simulink model "AutonomousScan"  (R2019a)
settings: Solver=FixedStepAuto  StartTime=0.0  StopTime=inf  FixedStep=0.001  RelTol=1e-3
libraries: dspnetwork x24, simulink_extras x3, etargetslib x1, dspmtrx3 x1, dspstat3 x1, simulink x1
(part 1 of 2)
settings Model: EnablePacing=on  Creator=jakub  LastModifiedBy=kirill
settings SolverCC: AutoInsertRateTranBlk=on
settings DataIOCC: ReturnWorkspaceOutputs=off
settings HardwareCC: ProdBitPerLong=64  ProdHWDeviceType=Intel->x86-64 (Linux 64)

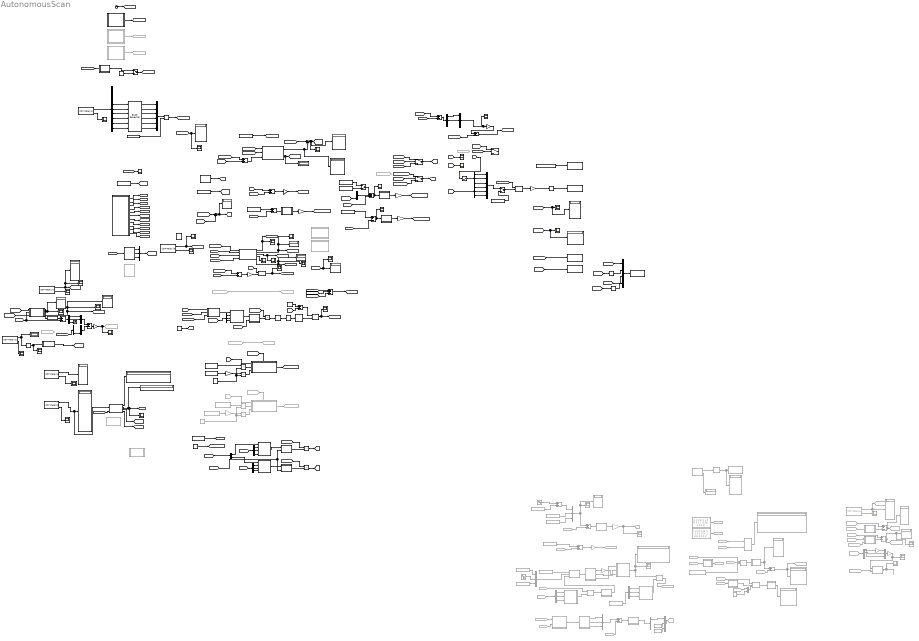
== system AutonomousScan ==
  note: Experimental RCM based on frame transforms - does not work. See ipad notes for details
  note: Experimental RCM based on screw axis - does not work
  note: Motoman - receiver (temp)
  note: Motoman Joint Position Control - depracated
  note: position control and trajectory generation
  note: force control
  note: y and z axes are zero'd twice (matlab function and matrix multiplication)
  note: transforms force sensor measured force to panda end effector frame to base frame
  note: Biasing sensor and panda position before moving - incorrect approach
  Add1 : Sum  Inputs=++-
  Add2 : Sum  Inputs=+-
  Add3 : Sum  Inputs=+-
  Byte Reversal : etargetslib/Byte Reversal  numInp=6
      settings: SourceProductName=MATLAB Coder  SourceProductBaseCode=ME
  Clock : Clock
  Constant1 : Constant  Commented=on  Value=[0.45;0;0.3]
  Constant10 : Constant  Value=[0.45;0;0.45]
  Constant11 : Constant  Value=0.25
  Constant12 : Constant  Value=[0;0;0]
  Constant13 : Constant  Value=2.25
  Constant14 : Constant  Value=-1.4
  Constant15 : Constant  Commented=on  Value=[0.25;0.25;0.25]
  Constant16 : Constant  Commented=on  Value=[0.5;0.5;0.5]
  Constant17 : Constant  Commented=on  Value=[0]
  Constant18 : Constant  Value=[0.553;0;0]
  Constant19 : Constant  Commented=on  Value=[0.5 0 0.06]
  Constant2 : Constant  Value=8.295632e-317  OutDataTypeStr=double
  Constant20 : Constant  Commented=on  Value=3.14
  Constant21 : Constant  Commented=on  Value=[0.5]
  Constant22 : Constant
  Constant23 : Constant  Value=1000000
  Constant24 : Constant  Value=[pi;0;-0.2]
  Constant25 : Constant  Commented=on  Value=[ 0.03]
  Constant26 : Constant  Commented=on  Value=[0]
  Constant27 : Constant  Commented=on  Value=[ 0]
  Constant28 : Constant  Commented=on  Value=[0;-pi;pi/2]
  Constant29 : Constant  Commented=on  Value=[0;0;0.02;1]
  Constant3 : Constant  Value=[0;0;0;0;0;0]
  Constant30 : Constant  Commented=on  Value=[1 0 0 0; 0 1 0 0; 0 0 1 -0.05; 0 0 0 1]
  Constant31 : Constant  Commented=on  Value=[1]
  Constant32 : Constant  Commented=on  Value=[1 0 0 0.45; 0 -1 0 0; 0 0 -1 0.3; 0 0 0 1]
  Constant33 : Constant  Value=[pi;0;pi/2-0.2]
  Constant34 : Constant  Value=[pi;0;-0.2]
  Constant35 : Constant  Value=[pi;0;-0.2]
  Constant4 : Constant  Value=[1 0 0; 0 1 0; 0 0 0]
  Constant5 : Constant  Commented=on  Value=[0]
  Constant6 : Constant  Value=[pi/2;0;pi]
  Constant7 : Constant  Commented=on  Value=1.5
  Constant8 : Constant  Value=[2.5;2.5;2.5]
  Constant9 : Constant  Value=[5;5;5]
  Degrees to Radians : simulink_extras/Transformations/Degrees to Radians
  Demux{1..2,4..5,7,12..13,15} (8 alike) : Demux  Outputs=3
  Demux10 : Demux  Commented=on  Outputs=7
  Demux11 : Demux  Outputs=9
  Demux3 : Demux  Outputs=2
  Demux6 : Demux  Commented=on  Outputs=3
  Demux8 : Demux  Commented=on  Outputs=3
  Demux9 : Demux  Commented=on  Outputs=3
  DerivOut1 : Scope
  Display{1..6,9..10,12,21..29} (18 alike) : Display
      Display2 settings: Decimation=4
      Display3 settings: Decimation=4
      Display4 settings: Decimation=4
  Display{7..8,11,13..20} (11 alike) : Display  Commented=on
      Display13 settings: Decimation=4
      Display14 settings: Decimation=4
      Display16 settings: Decimation=4
  Divide4 : Product  Inputs=*/  OutDataTypeStr=double
  From1 : From  Commented=on  GotoTag=M_cart
  From12 : From  Commented=on  GotoTag=admission_vel_cart
  From26 : From  Commented=on  GotoTag=bias_good
  From30 : From  Commented=on  GotoTag=admission_vel_rot
  From47 : From  Commented=on  GotoTag=vel_rot
  From48 : From  Commented=on  GotoTag=panda_pos_biased
  From49 : From  Commented=on  GotoTag=sensor
  From50 : From  Commented=on  GotoTag=sensor
  From51 : From  Commented=on  GotoTag=scan_complete
  From{52..53,57,68,70,74} (6 alike) : From  Commented=on  GotoTag=panda_pos
  From55 : From  Commented=on  GotoTag=panda_rpy
  From58 : From  Commented=on  GotoTag=panda_so3
  From60 : From  Commented=on  GotoTag=axia_ft
  From61 : From  Commented=on  GotoTag=rot_des_bf2
  From62 : From  Commented=on  GotoTag=panda_so3
  From63 : From  Commented=on  GotoTag=panda_so3
  From64 : From  Commented=on  GotoTag=panda_rpy
  From65 : From  Commented=on  GotoTag=T_B_EE
  From67 : From  Commented=on  GotoTag=T_U_EE
  From71 : From  Commented=on  GotoTag=invU
  From72 : From  Commented=on  GotoTag=T_U_EE
  From73 : From  Commented=on  GotoTag=T_B_EE
  From75 : From  Commented=on  GotoTag=sensor_biased
  From80 : From  Commented=on  GotoTag=bias_good
  From90 : From  Commented=on  GotoTag=admission_control
  Gain : Gain  Gain=3.0
  Gain1 : Gain  Gain=2.5
  Gain10 : Gain  Commented=on  Gain=-1
  Gain11 : Gain  Gain=3.0
  Gain{4..5,12,14} (4 alike) : Gain  Gain=0.5
  Gain13 : Gain  Gain=3.0
  Gain2 : Gain  Gain=1.0
  Gain3 : Gain  Commented=on  Gain=2.75
  Gain6 : Gain  Commented=on  Gain=0.5
  Gain7 : Gain  Commented=on  Gain=3.0
  Gain8 : Gain  Commented=on  Gain=0
  Gain9 : Gain  Commented=on  Gain=0.1
  Goto13 : Goto  Commented=on  GotoTag=admission_vel_rot
  Goto17 : Goto  Commented=on  GotoTag=admission_control
  Goto27 : Goto  Commented=on  GotoTag=sensor
  Goto28 : Goto  Commented=on  GotoTag=vel_rot
  Goto29 : Goto  Commented=on  GotoTag=sensor_biased
  Goto30 : Goto  Commented=on  GotoTag=panda_pos_biased
  Goto31 : Goto  Commented=on  GotoTag=V_cart_2
  Goto32 : Goto  Commented=on  GotoTag=vel_rot
  Goto33 : Goto  Commented=on  GotoTag=vel_tran_temp
  Goto34 : Goto  Commented=on  GotoTag=rot_des_bf2
  Goto36 : Goto  Commented=on  GotoTag=vel_rot
  Goto41 : Goto  Commented=on  GotoTag=vel_tran_temp
  Goto42 : Goto  Commented=on  GotoTag=panda_ijac
  Goto43 : Goto  Commented=on  GotoTag=panda_state
  Goto47 : Goto  Commented=on  GotoTag=invU
  Goto48 : Goto  Commented=on  GotoTag=T_U_EE
  Goto57 : Goto  Commented=on  GotoTag=T_B_EE
  Identity Matrix : dspmtrx3/Identity Matrix  Inherit=off  N=3  Ts=1  dataType=double  isSigned=on  wordLen=16  udDataType=sfix(16)  fracBitsMode=Best precision  numFracBits=15  OutDataTypeStr=double  LastOutDataTypeStr=double
      settings: SourceProductName=DSP System Toolbox
  MATLAB Function : MATLAB Function  TreatAsAtomicUnit=on
  MATLAB Function1 : MATLAB Function  TreatAsAtomicUnit=on
  MATLAB Function10 : MATLAB Function  Commented=on  TreatAsAtomicUnit=on
  MATLAB Function11 : MATLAB Function  Commented=on  TreatAsAtomicUnit=on
  MATLAB Function12 : MATLAB Function  Commented=on  TreatAsAtomicUnit=on
  MATLAB Function13 : MATLAB Function  Commented=on  TreatAsAtomicUnit=on
  MATLAB Function14 : MATLAB Function  Commented=on  TreatAsAtomicUnit=on
  MATLAB Function15 : MATLAB Function  Commented=on  TreatAsAtomicUnit=on
  MATLAB Function16 : MATLAB Function  Commented=on  TreatAsAtomicUnit=on
  MATLAB Function17 : MATLAB Function  Commented=on  TreatAsAtomicUnit=on
  MATLAB Function18 : MATLAB Function  Commented=on  TreatAsAtomicUnit=on
  MATLAB Function19 : MATLAB Function  Commented=on  TreatAsAtomicUnit=on
  MATLAB Function2 : MATLAB Function  TreatAsAtomicUnit=on
  MATLAB Function20 : MATLAB Function  Commented=on  TreatAsAtomicUnit=on
  MATLAB Function21 : MATLAB Function  Commented=on  TreatAsAtomicUnit=on
  MATLAB Function22 : MATLAB Function  Commented=on  TreatAsAtomicUnit=on
  MATLAB Function23 : MATLAB Function  Commented=on  TreatAsAtomicUnit=on
  MATLAB Function24 : MATLAB Function  Commented=on  TreatAsAtomicUnit=on
  MATLAB Function25 : MATLAB Function  Commented=on  TreatAsAtomicUnit=on
  MATLAB Function26 : MATLAB Function  TreatAsAtomicUnit=on
  MATLAB Function27 : MATLAB Function  TreatAsAtomicUnit=on
  MATLAB Function28 : MATLAB Function  TreatAsAtomicUnit=on
  MATLAB Function29 : MATLAB Function  Commented=on  TreatAsAtomicUnit=on
  MATLAB Function3 : MATLAB Function  TreatAsAtomicUnit=on
  MATLAB Function30 : MATLAB Function  TreatAsAtomicUnit=on
  MATLAB Function31 : MATLAB Function  Commented=on  TreatAsAtomicUnit=on
  MATLAB Function32 : MATLAB Function  TreatAsAtomicUnit=on
  MATLAB Function33 : MATLAB Function  TreatAsAtomicUnit=on
  MATLAB Function34 : MATLAB Function  TreatAsAtomicUnit=on
  MATLAB Function4 : MATLAB Function  TreatAsAtomicUnit=on
  MATLAB Function5 : MATLAB Function  TreatAsAtomicUnit=on
  MATLAB Function6 : MATLAB Function  TreatAsAtomicUnit=on
  MATLAB Function7 : MATLAB Function  TreatAsAtomicUnit=on
  MATLAB Function8 : MATLAB Function  TreatAsAtomicUnit=on
  MATLAB Function9 : MATLAB Function  Commented=on  TreatAsAtomicUnit=on
  Manual Switch : ManualSwitch
  Manual Switch1 : ManualSwitch  CurrentSetting=0
  Matrix Multiply : Product  Multiplication=Matrix(*)
  Matrix Multiply1 : Product  Multiplication=Matrix(*)
  Matrix Multiply2 : Product  Multiplication=Matrix(*)
  Matrix Multiply3 : Product  Commented=on  Multiplication=Matrix(*)
  Matrix Multiply4 : Product  Commented=on  Multiplication=Matrix(*)
  Matrix Multiply5 : Product  Commented=on  Inputs=3  Multiplication=Matrix(*)
  Matrix Multiply6 : Product  Commented=on  Inputs=3  Multiplication=Matrix(*)
  Moving Average : dspstat3/Moving Average  Method=Sliding window  ForgettingFactorPort=off  SpecifyWindowLength=on  WindowLength=800  ForgettingFactor=0.9  SimulateUsing=Code generation
  Mux : Mux  Inputs=6
  Mux{1..4,6} (5 alike) : Mux  Commented=on  Inputs=3
  Mux10 : Mux  Inputs=6
  Mux11 : Mux
  Mux{7..9,12,14} (5 alike) : Mux  Inputs=3
  Mux5 : Mux  Commented=on  Inputs=2
  NetworkPacket : Scope
  New Phantom : MATLAB Function  TreatAsAtomicUnit=on
  PID Controller2 : simulink/Continuous/PID Controller  Controller=PID  Form=Parallel  TimeDomain=Continuous-time  SampleTime=-1  IntegratorMethod=Forward Euler  FilterMethod=Forward Euler  ControllerParametersSource=internal  P=0.2  I=0  D=0.1  UseFilter=on  N=100  TunerSelectOption=Transfer Function Based (PID Tuner App)  InitialConditionSource=internal  InitialConditionForIntegrator=0  InitialConditionForFilter=0  DifferentiatorICPrevScaledInput=0  ExternalReset=none  TrackingMode=off  Kt=1  LimitOutput=off  UpperSaturationLimit=inf  LowerSaturationLimit=-inf  LinearizeAsGain=on  AntiWindupMode=none  Kb=1  POutMin=[]  POutMax=[]  IOutMin=[]  IOutMax=[]  DOutMin=[]  DOutMax=[]  NOutMin=[]  NOutMax=[]  SumOutMin=[]  SumOutMax=[]  SaturationOutMin=[]  SaturationOutMax=[]  PParamMin=[]  PParamMax=[]  IParamMin=[]  IParamMax=[]  DParamMin=[]  DParamMax=[]  NParamMin=[]  NParamMax=[]  KbParamMin=[]  KbParamMax=[]  KtParamMin=[]  KtParamMax=[]  KbOutMin=[]  KbOutMax=[]  KtOutMin=[]  KtOutMax=[]  IntegratorOutMin=[]  IntegratorOutMax=[]  FilterOutMin=[]  FilterOutMax=[]  SumI1OutMin=[]  SumI1OutMax=[]  SumI2OutMin=[]  SumI2OutMax=[]  SumI3OutMin=[]  SumI3OutMax=[]  SumI4OutMin=[]  SumI4OutMax=[]  SumDOutMin=[]  SumDOutMax=[]  DifferentiatorOutMin=[]  DifferentiatorOutMax=[]  FilterDiffOutCoefMin=[]  FilterDiffOutCoefMax=[]  ReciprocalOutMin=[]  ReciprocalOutMax=[]  SumDenOutMin=[]  SumDenOutMax=[]  SumNumOutMin=[]  SumNumOutMax=[]  DivideOutMin=[]  DivideOutMax=[]  IntegratorContinuousStateAttributes=''  IntegratorStateMustResolveToSignalObject=off  IntegratorRTWStateStorageClass=Auto  FilterContinuousStateAttributes=''  FilterStateMustResolveToSignalObject=off  FilterRTWStateStorageClass=Auto  ParallelPVariant=InternalParameters  IdealPVariant=Disabled  IVariant=InternalParameters  DVariant=InternalParameters  IntegratorVariant=Continuous  SatVariant=Disabled  AWVariant=Passthrough  PCopyVariant=Disabled  TRVariant=Disabled  FdbkBlocksVariant=Forward  IdealPFdbkVariant=Disabled  SatFdbkVariant=Disabled  DerivativeFilterVariant=ContFilter  NVariant=InternalParameters  NCopyVariant=Disabled  FilterICVariant=InternalICsFilter  IntegratorICVariant=InternalICs  ExternalResetVariant=Disabled  TRSumVariant=Passthrough  SumFdbkVariant=Disabled  SumVariant=Sum_PID
  PandaPosition : Scope
  PandaRotation : Scope
  PandaRotation1 : Scope  Commented=on
  Panda_inv_jac_receive : Subsystem  Commented=on
  Panda_inv_jac_receive1 : Subsystem  Commented=on
  Product{,1,4..6} (5 alike) : Product
  Product2 : Product  Commented=on
  Product3 : Product  Commented=on
  Radians to Degrees : simulink_extras/Transformations/Radians to Degrees
  Radians to Degrees1 : simulink_extras/Transformations/Radians to Degrees
  Rate Limiter1 : RateLimiter  RisingSlewLimit=2.0  FallingSlewLimit=-2.0  SampleTimeMode=inherited
  Rate Limiter3 : RateLimiter  RisingSlewLimit=0.15  FallingSlewLimit=-0.15  SampleTimeMode=inherited
  Rate Transition : RateTransition  OutPortSampleTime=0.01
  Rate Transition1 : RateTransition  Commented=on  OutPortSampleTime=2
  STOP_SWITCH1 : ManualSwitch
  Saturation : Saturate  UpperLimit=0.1  LowerLimit=-0.1
  Scope{,1..9,12,17..23,25..26,28..29} (22 alike) : Scope
  Scope{10..11,13..16} (6 alike) : Scope  Commented=on
  Sine Wave : Sin  Commented=on  Amplitude=0.4  Frequency=3  SampleTime=0
  Sine Wave1 : Sin  Commented=on  Amplitude=0.05  Frequency=3  SampleTime=0
  Subtract{1..4,13,15..16} (7 alike) : Sum  Inputs=+-
  Subtract10 : Sum  Commented=on
  Subtract{5..8,11..12} (6 alike) : Sum  Commented=on  Inputs=+-
  Subtract14 : Sum  Inputs=+--
  Subtract9 : Sum
  Sum : Sum  Inputs=|+-
  Sum2 : Sum  Inputs=|++
  Switch1 : Switch  Criteria=u2 > Threshold
  Switch2 : Switch  Criteria=u2 > Threshold
  Switch3 : Switch  Criteria=u2 > Threshold
  Terminator : Terminator
  Trajectory Generation (works) : MATLAB Function  Commented=on  TreatAsAtomicUnit=on
  Trajectory Generation1 : MATLAB Function  Commented=on  TreatAsAtomicUnit=on
  UDP Receive1 : dspnetwork/UDP Receive  localURL='0.0.0.0'  localPort=49154  remoteURL='192.168.0.13'  remotePort=-1  recvBufferSize=36  dims=9  signalDatatype=int32  isComplex=off  isVarSize=off  showBlockingTime=off  blockingTime=0  sampletime=0.001  blockPlatform=[]
      settings: SourceProductName=Simulink
  UDP Receive2 : dspnetwork/UDP Receive  localURL='0.0.0.0'  localPort=25010  remoteURL='10.1.38.120'  remotePort=-1  recvBufferSize=8192  dims=1  signalDatatype=double  isComplex=off  isVarSize=off  showBlockingTime=off  blockingTime=0  sampletime=0.001  blockPlatform=[]
      settings: SourceProductName=Simulink
  UDP Receive3 : dspnetwork/UDP Receive  Commented=on  localURL='0.0.0.0'  localPort=1502  remoteURL='10.1.38.120'  remotePort=-1  recvBufferSize=8192  dims=7  signalDatatype=double  isComplex=off  isVarSize=off  showBlockingTime=off  blockingTime=0  sampletime=0.001  blockPlatform=[]
      settings: SourceProductName=Simulink
  UDP Receive4 : dspnetwork/UDP Receive  localURL='0.0.0.0'  localPort=30011  remoteURL='0.0.0.0'  remotePort=-1  recvBufferSize=8192  dims=7  signalDatatype=double  isComplex=off  isVarSize=off  showBlockingTime=off  blockingTime=0  sampletime=0.1  blockPlatform=[]
      settings: SourceProductName=Simulink
  UDP Receive5 : dspnetwork/UDP Receive  localURL='0.0.0.0'  localPort=1502  remoteURL='192.168.100.101'  remotePort=-1  recvBufferSize=8192  dims=7  signalDatatype=double  isComplex=off  isVarSize=off  showBlockingTime=off  blockingTime=0  sampletime=0.001  blockPlatform=[]
      settings: SourceProductName=Simulink
  UDP Receive6 : dspnetwork/UDP Receive  localURL='0.0.0.0'  localPort=30015  remoteURL='0.0.0.0'  remotePort=-1  recvBufferSize=8192  dims=15  signalDatatype=double  isComplex=off  isVarSize=off  showBlockingTime=off  blockingTime=0  sampletime=0.1  blockPlatform=[]
      settings: SourceProductName=Simulink
  UDP Receive7 : dspnetwork/UDP Receive  localURL='0.0.0.0'  localPort=1508  remoteURL='10.1.38.120'  remotePort=-1  recvBufferSize=8192  dims=1  signalDatatype=double  isComplex=off  isVarSize=off  showBlockingTime=off  blockingTime=0  sampletime=0.001  blockPlatform=[]
      settings: SourceProductName=Simulink
  UDP Send1 : dspnetwork/UDP Send  remoteURL='127.0.0.1'  remotePort=39474  localURL='0.0.0.0'  localPortSource=Automatically determine  localPort=48000  sampletime=-1  blockPlatform=[]  separateLengthPort=0
      settings: SourceProductName=Simulink
  UDP Send2 : dspnetwork/UDP Send  remoteURL='10.1.38.120'  remotePort=25002  localURL='0.0.0.0'  localPortSource=Specify via dialog  localPort=25004  sampletime=-1  blockPlatform=[]  separateLengthPort=0
      settings: SourceProductName=Simulink
  UDP Send3 : dspnetwork/UDP Send  remoteURL='10.1.38.120'  remotePort=25006  localURL='0.0.0.0'  localPortSource=Specify via dialog  localPort=25008  sampletime=-1  blockPlatform=[]  separateLengthPort=0
      settings: SourceProductName=Simulink
  UDP Send4 : dspnetwork/UDP Send  remoteURL='192.168.0.13'  remotePort=49152  localURL='0.0.0.0'  localPortSource=Specify via dialog  localPort=49154  sampletime=-1  blockPlatform=[]  separateLengthPort=0
      settings: SourceProductName=Simulink
  UDP Send5 : dspnetwork/UDP Send  Commented=on  remoteURL='127.0.0.1'  remotePort=39575  localURL='0.0.0.0'  localPortSource=Automatically determine  localPort=48000  sampletime=-1  blockPlatform=[]  separateLengthPort=0
      settings: SourceProductName=Simulink
  UDP Send6 : dspnetwork/UDP Send  remoteURL='10.1.38.120'  remotePort=35000  localURL='0.0.0.0'  localPortSource=Specify via dialog  localPort=25008  sampletime=-1  blockPlatform=[]  separateLengthPort=0
      settings: SourceProductName=Simulink
  Velocity Controller1 : Subsystem
  Velocity Controller2 : Subsystem  Commented=on
  VelocityOut{,1..4} (5 alike) : Scope
  in general1 : MATLAB Function  TreatAsAtomicUnit=on
  in general2 : MATLAB Function  Commented=on  TreatAsAtomicUnit=on
  in general3 : MATLAB Function  Commented=on  TreatAsAtomicUnit=on
  in general4 : MATLAB Function  Commented=on  TreatAsAtomicUnit=on
  joy_state_receive1 : Subsystem
  panda_data_receive : Subsystem
  wires:
  Demux2/1 -> Mux/1
  Demux1/2 -> Mux/5
  Demux1/1 -> Mux/4
  Demux2/2 -> Mux/2
  Demux1/3 -> Mux/6
  Demux2/3 -> Mux/3
  [V_rot] -> Demux1/1
  Constant18/1 -> [P_tissue]
  joy_state_receive1/1("joy_state ") -> [joy_state]
  Panda_inv_jac_receive1/1(panda_state) -> Goto43/1
  [joy_state] -> MATLAB Function33/1(u)
  MATLAB Function33/1(stop) -> STOP_SWITCH1/1
  Panda_inv_jac_receive/1(inverse_jacobian) -> Goto42/1
  STOP_SWITCH1/1 -> [stop_manual]
  Constant22/1 -> STOP_SWITCH1/2
  in general1/1(grad) -> Mux7/1
  in general1/2(brad) -> Mux7/2
  in general1/3(arad) -> Mux7/3
  Mux7/1 -> [panda_rpy]
  [panda_ijac] -> Matrix Multiply/1
  Clock/1 -> [sim_time]
  UDP Receive1/2 -> NetworkPacket/1
  Byte Reversal/4 -> Mux10/4
  Divide4/1 -> [axia_force]
  Byte Reversal/2 -> Mux10/2
  Constant23/1 -> Divide4/2
  Demux11/7 -> Byte Reversal/4
  Mux10/1 -> Divide4/1
  Byte Reversal/1 -> Mux10/1
  Demux11/5 -> Byte Reversal/2
  UDP Receive1/1 -> Demux11/1
  Demux11/6 -> Byte Reversal/3
  Byte Reversal/3 -> Mux10/3
  Demux11/9 -> Byte Reversal/6
  Demux11/8 -> Byte Reversal/5
  Demux11/4 -> Byte Reversal/1
  Byte Reversal/5 -> Mux10/5
  Byte Reversal/6 -> Mux10/6
  [panda_pos] -> Display4/1, PandaPosition/1
  [V_cart] -> VelocityOut/1
  panda_data_receive/9(panda_tau) -> [panda_tau]
  panda_data_receive/4(panda_force) -> [panda_force]
  panda_data_receive/2(panda_pos) -> [panda_pos]
  panda_data_receive/10(panda_state) -> [panda_state]
  panda_data_receive/3(panda_so3) -> [panda_so3]
  panda_data_receive/7(inverse_jacobian) -> [panda_ijac]
  panda_data_receive/6(panda_dq) -> [panda_dq]
  panda_data_receive/1(ros_time) -> [ros_time]
  panda_data_receive/5(panda_q) -> [panda_q]
  panda_data_receive/8(jacobian) -> [panda_jac]
  [panda_rpy] -> Display3/1, PandaRotation/1
  Constant24/1 -> Subtract3/1
  [panda_rpy] -> Subtract3/2
  panda_data_receive/11(networkVals) -> [networkVals]
  [p_des] -> Subtract1/1
  Gain2/1 -> Rate Limiter1/1
  Matrix Multiply/1 -> Gain2/1
  Constant2/1 -> UDP Send4/1
  Subtract1/1 -> Gain/1
  [panda_pos] -> Subtract1/2
  [panda_ijac] -> DerivOut1/1
  Sum2/1 -> Display1/1, [p_des]
  [probe_offset] -> Sum2/2
  Saturation/1 -> Demux2/1
  Constant12/1 -> [probe_offset]
  Mux/1 -> Manual Switch/1
  Manual Switch/1 -> Matrix Multiply/2
  Constant3/1 -> Manual Switch/2
  [axia_force] -> Scope5/1, Display2/1
  MATLAB Function5/1(bias) -> Display6/1, Sum/2
  [axia_force] -> Sum/1
  Sum/1 -> Scope/1, Display10/1, [axia_biased]
  MATLAB Function5/2(forceBiasGood) -> Display5/1, [bias_good]
  Constant10/1 -> [p_bias]
  [axia_force] -> MATLAB Function5/1(forceMeasure)
  [p_bias] -> Subtract9/1
  Constant11/1 -> [f_scale_factor]
  MATLAB Function8/1(x_rot) -> Product5/2
  MATLAB Function/1(x_rot) -> Product4/2
  Demux3/2 -> MATLAB Function7/1(X)
  Demux4/2 -> MATLAB Function7/3(brad)
  Demux5/3 -> MATLAB Function6/4(grad)
  Demux3/1 -> MATLAB Function6/1(X)
  [axia_ft] -> Demux5/1
  Demux4/3 -> MATLAB Function7/4(grad)
  Demux4/1 -> MATLAB Function7/2(arad)
  [axia_ft] -> Demux4/1
  MATLAB Function6/1(X_t) -> MATLAB Function/1(x)
  [f_scale_factor] -> Product5/1
  [f_scale_factor] -> Product4/1
  Product4/1 -> [F_cart]
  MATLAB Function7/1(X_t) -> MATLAB Function8/1(x)
  [panda_so3] -> MATLAB Function/2(R), MATLAB Function8/2(R)
  Demux5/2 -> MATLAB Function6/3(brad)
  Product5/1 -> [M_cart]
  Constant6/1 -> [axia_ft]
  Gain1/1 -> Product1/1
  Constant8/1 -> Product/1
  Constant9/1 -> Gain1/1
  Product/1 -> Velocity Controller1/2(m)
  Product1/1 -> Velocity Controller1/3(c)
  [F_cart] -> Velocity Controller1/1(F_Total)
  [bias_good] -> Switch1/2
  [p_bias] -> Sum2/1
  Demux5/1 -> MATLAB Function6/2(arad)
  Constant13/1 -> Product1/2, Product/2
  [V_rot] -> VelocityOut1/1
  Gain3/1 -> Product3/1
  Product3/1 -> Velocity Controller2/3(c)
  Constant7/1 -> Product2/2, Product3/2
  Constant16/1 -> Gain3/1
  Product2/1 -> Velocity Controller2/2(m)
  Constant15/1 -> Product2/1
  From1/1 -> Velocity Controller2/1(M_Total)
  [bias_good] -> Switch3/2
  Switch3/1 -> [V_rot]
  [bias_good] -> Velocity Controller1/Enable
  [initial_vel_rot] -> Switch3/3
  From26/1 -> Velocity Controller2/Enable
  Velocity Controller2/1(Vel_Rot) -> Goto13/1
  [initial_vel_tran] -> Switch1/3
  [vel_rot_scan] -> Switch3/1
  Rate Limiter1/1 -> UDP Send1/1
  From30/1 -> Goto28/1
  [vel_tran] -> Switch1/1
  Switch1/1 -> [V_cart]
  Subtract3/1 -> MATLAB Function1/1(u)
  Gain/1 -> [initial_vel_tran]
  MATLAB Function1/1(y) -> Gain5/1
  Gain5/1 -> [initial_vel_rot]
  [panda_pos] -> Subtract2/2
  Constant14/1 -> [fdes_z]
  [axia_biased] -> Demux3/1
  Velocity Controller1/1(Vel_Cart) -> [admission_vel_cart]
  [fdes_z] -> MATLAB Function3/1(f_des)
  [axia_biased] -> MATLAB Function3/2(f_act)
  [bias_good] -> MATLAB Function3/3(bias_good)
  Demux7/1 -> MATLAB Function4/2(arad)
  Demux7/2 -> MATLAB Function4/3(brad)
  [panda_so3] -> MATLAB Function2/2(R)
  MATLAB Function4/1(X_t) -> MATLAB Function2/1(x)
  MATLAB Function2/1(x_rot) -> Product6/2
  Demux7/3 -> MATLAB Function4/4(grad)
  [axia_ft] -> Demux7/1
  MATLAB Function3/1(f_err) -> MATLAB Function4/1(X)
  [f_scale_factor] -> Product6/1
  PID Controller2/1 -> Rate Limiter3/1
  Matrix Multiply1/1 -> Scope4/1, [pos_control]
  Constant4/1 -> [S]
  Identity Matrix/1 -> Subtract4/1
  [S] -> Subtract4/2
  Subtract4/1 -> Matrix Multiply2/1
  Product6/1 -> PID Controller2/1
  Rate Limiter3/1 -> Moving Average/1
  [S] -> Matrix Multiply1/1
  Matrix Multiply2/1 -> [force_control], Scope2/1
  Moving Average/1 -> Matrix Multiply2/2
  From12/1 -> Goto17/1
  [admission_control] -> Add1/2
  [force_control] -> Add1/3
  [pos_des] -> Subtract2/1
  [panda_pos] -> New Phantom/2(current_pos)
  New Phantom/1(pos_des) -> [pos_des], Scope1/1
  New Phantom/2(record_data) -> Scope6/1, Display9/1, [record_data]
  [axia_biased] -> New Phantom/3(measured_force)
  [bias_good] -> New Phantom/4(bias_good)
  Subtract2/1 -> Gain4/1
  [shutter] -> UDP Send2/1
  [panda_pos] -> UDP Send3/1
  Gain4/1 -> Matrix Multiply1/2
  New Phantom/3(shutter) -> Scope3/1, [shutter]
  UDP Receive2/2 -> Scope7/1
  [shutter_fb] -> New Phantom/1(shutter_fb)
  New Phantom/4(pnts) -> Scope9/1
  UDP Receive4/1 -> Display12/1
  UDP Receive4/2 -> Scope12/1
  Rate Transition1/1 -> Display13/1, UDP Send5/1
  MATLAB Function12/1(y) -> Rate Transition1/1
  MATLAB Function12/2(limit) -> Display14/1
  Subtract10/1 -> Mux1/1
  Constant5/1 -> Mux1/2
  Constant17/1 -> Mux1/3
  MATLAB Function13/1(y) -> Gain6/1
  Gain6/1 -> Scope14/1, Goto32/1
  [panda_pos] -> MATLAB Function5/2(currentPos)
  Subtract9/1 -> MATLAB Function5/3(desiredPos)
  [probe_offset] -> Subtract9/2
  Sine Wave/1 -> Subtract10/1
  Constant20/1 -> Subtract10/2
  Subtract7/1 -> MATLAB Function13/1(u)
  Mux1/1 -> Scope13/1, Display17/1, Subtract7/1
  From55/1 -> Subtract7/2
  [panda_so3] -> in general1/1(R)
  Constant1/1 -> Subtract11/1
  Subtract11/1 -> Gain7/1
  From57/1 -> Subtract11/2
  Gain7/1 -> Goto33/1
  Constant19/1 -> MATLAB Function14/1(rcm)
  Mux3/1 -> MATLAB Function14/2(tip)
  MATLAB Function14/1(rotmat) -> in general3/1(R)
  in general3/1(grad) -> Gain8/1
  in general3/2(brad) -> MATLAB Function15/2(brad)
  in general3/3(arad) -> MATLAB Function15/1(arad)
  Gain8/1 -> MATLAB Function15/3(grad)
  From60/1 -> Demux6/1
  From58/1 -> Matrix Multiply3/1
  MATLAB Function16/1(R) -> Matrix Multiply3/2
  Matrix Multiply3/1 -> MATLAB Function17/1(u)
  MATLAB Function17/1(y) -> MATLAB Function14/3(currentZ)
  Constant28/1 -> Demux8/1
  MATLAB Function15/1(R) -> Display16/1, PandaRotation1/1, Matrix Multiply4/1
  MATLAB Function18/1(R) -> Matrix Multiply4/2
  Matrix Multiply4/1 -> Goto34/1
  From61/1 -> MATLAB Function19/1(R_des)
  From63/1 -> MATLAB Function19/2(R_i)
  MATLAB Function19/1(R_err) -> in general4/1(R)
  in general4/1(grad) -> Mux2/1
  in general4/2(brad) -> Mux2/2
  in general4/3(arad) -> Mux2/3
  Mux2/1 -> Subtract12/1
  From64/1 -> Subtract12/2
  Subtract12/1 -> MATLAB Function20/1(u)
  Sine Wave1/1 -> Mux3/2
  Constant25/1 -> Mux3/3
  Constant21/1 -> Mux3/1
  MATLAB Function20/1(y) -> Demux9/1
  Constant27/1 -> Mux4/2
  Constant26/1 -> Mux4/3
  Demux9/1 -> Mux4/1
  Mux4/1 -> Goto36/1
  Demux8/1 -> MATLAB Function18/1(arad)
  Demux8/2 -> MATLAB Function18/2(brad)
  Demux8/3 -> MATLAB Function18/3(grad)
  Demux6/1 -> MATLAB Function16/1(arad)
  Demux6/2 -> MATLAB Function16/2(brad)
  Demux6/3 -> MATLAB Function16/3(grad)
  From62/1 -> MATLAB Function21/1(R)
  From70/1 -> MATLAB Function21/2(P)
  MATLAB Function21/1(T) -> Display15/1
  Matrix Multiply5/1 -> MATLAB Function22/1(u)
  From67/1 -> MATLAB Function24/1(u)
  Constant29/1 -> Matrix Multiply5/3
  From65/1 -> Matrix Multiply5/1
  MATLAB Function24/1(y) -> Goto47/1
  From71/1 -> Matrix Multiply5/2
  Subtract8/1 -> Display19/1, Goto41/1
  MATLAB Function22/1(y) -> Display18/1, Subtract8/1
  MATLAB Function25/1(y) -> Display20/1
  Constant30/1 -> Goto48/1
  From72/1 -> Matrix Multiply6/1
  MATLAB Function23/1(y) -> Matrix Multiply6/2
  From73/1 -> MATLAB Function23/1(u)
  Matrix Multiply6/1 -> MATLAB Function25/1(u)
  From68/1 -> Mux5/1
  Constant31/1 -> Mux5/2
  Mux5/1 -> Matrix Multiply6/3
  From74/1 -> Subtract8/2
  Constant32/1 -> Goto57/1
  [bias_good] -> Switch2/2
  New Phantom/5(scan_complete) -> [scan_complete], Display26/1, Scope23/1
  MATLAB Function26/1(pandaDes) -> Display21/1, Scope17/1, MATLAB Function28/1(pandaPos)
  [sensor] -> MATLAB Function26/1(sensor)
  [panda_pos] -> MATLAB Function26/2(pandaCurrent), Add3/2
  Demux12/1 -> Mux8/1
  Demux12/2 -> Mux8/2
  Demux12/3 -> Terminator/1
  Mux8/1 -> Add2/1
  [force_control] -> Demux13/1
  Demux13/3 -> Mux9/3
  Mux9/1 -> Add2/2
  Add3/1 -> Demux12/1
  Gain11/1 -> Scope18/1, Goto31/1
  Add2/1 -> Gain11/1
  UDP Receive5/2 -> Scope19/1
  UDP Receive5/1 -> Scope28/1, Display23/1, [sensor]
  From50/1 -> Subtract5/1
  MATLAB Function10/1(y) -> Subtract5/2
  From49/1 -> MATLAB Function10/1(sensor)
  From48/1 -> MATLAB Function9/2(panda_pos)
  UDP Receive3/2 -> Scope10/1
  Gain9/1 -> MATLAB Function9/1(u), Scope15/1
  Subtract5/1 -> Display8/1, Goto29/1
  Demux10/3 -> Mux6/2
  From52/1 -> MATLAB Function11/1(panda_pos)
  From75/1 -> Demux10/1
  Mux6/1 -> Gain9/1
  Demux10/1 -> Mux6/3
  MATLAB Function11/1(y) -> Subtract6/2
  Demux10/2 -> Gain10/1
  From53/1 -> Subtract6/1
  UDP Receive3/1 -> Goto27/1, Display7/1
  From80/1 -> MATLAB Function11/2(intraop)
  Gain10/1 -> Mux6/1
  Subtract6/1 -> Scope16/1, Display11/1, Goto30/1
  MATLAB Function9/1(V_cart_2) -> Scope11/1
  [panda_pos] -> Mux11/1
  Mux11/1 -> UDP Send6/1
  [panda_rpy] -> Radians to Degrees/1
  UDP Receive6/2 -> Scope20/1
  MATLAB Function27/1(y) -> Gain12/1
  Subtract14/1 -> VelocityOut2/1, MATLAB Function27/1(u)
  [panda_rpy] -> Subtract14/3
  Constant34/1 -> Manual Switch1/2
  Mux12/1 -> Subtract14/2
  [rotZ] -> Mux12/3
  UDP Receive7/1 -> Degrees to Radians/1, Display25/1
  UDP Receive7/2 -> Scope21/1
  Degrees to Radians/1 -> MATLAB Function30/1(input), Scope22/1
  [V_cart_2] -> Switch2/1
  Gain12/1 -> [vel_rot]
  [motoman_pos] -> Mux11/3
  Radians to Degrees/1 -> Mux11/2
  [panda_pos] -> Scope25/1, Display22/1
  Constant33/1 -> Manual Switch1/1
  Manual Switch1/1 -> Subtract14/1
  [rotZ] -> MATLAB Function26/3(rotZ)
  MATLAB Function28/1(pandaDes) -> Add3/1
  UDP Receive6/1 -> MATLAB Function32/1(message), Display24/1
  MATLAB Function32/2(needletip_pos) -> Display28/1, Scope26/1, [test_pos]
  Demux15/1 -> Mux14/1
  Demux15/2 -> Mux14/2
  MATLAB Function26/3(sensorCurrent) -> Scope29/1, Display29/1, [sensorCurrent]
  MATLAB Function30/1(rotZ) -> [rotZ]
  [sensorCurrent] -> MATLAB Function32/2(sensor)
  MATLAB Function32/1(motoman_transform) -> Display27/1
  Mux14/1 -> VelocityOut3/1, Gain13/1
  [force_control] -> Subtract13/2
  Gain13/1 -> Subtract13/1
  Subtract13/1 -> [V_cart_2]
  [test_pos] -> Subtract15/1
  [panda_pos] -> Subtract15/2
  Subtract15/1 -> Demux15/1
  [panda_rpy] -> Subtract16/2
  Subtract16/1 -> VelocityOut4/1, MATLAB Function34/1(u)
  Gain14/1 -> [vel_rot_scan]
  MATLAB Function34/1(y) -> Gain14/1
  Constant35/1 -> Subtract16/1
  [V_cart] -> Saturation/1
  MATLAB Function32/3(motoman_pos) -> [motoman_pos]
  UDP Receive2/1 -> Scope8/1, [shutter_fb]
  MATLAB Function32/4(motoman_rpy) -> [motoman_rpy]
  [motoman_rpy] -> Radians to Degrees1/1
  Radians to Degrees1/1 -> Mux11/4
  [pos_control] -> Add1/1
  Add1/1 -> [vel_tran]

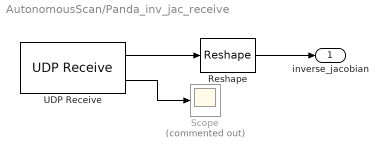
== system AutonomousScan/Panda_inv_jac_receive ==
  Reshape : Reshape  OutputDimensionality=Customize  OutputDimensions=[7,6]
  Scope : Scope  Commented=on
  UDP Receive : dspnetwork/UDP Receive  localURL='0.0.0.0'  localPort=30005  remoteURL='0.0.0.0'  remotePort=-1  recvBufferSize=3360  dims=42  signalDatatype=double  isComplex=off  isVarSize=off  showBlockingTime=off  blockingTime=0  sampletime=0.001  blockPlatform=[]
      settings: SourceProductName=Simulink
  inverse_jacobian : Outport
  wires:
  UDP Receive/2 -> Scope/1
  UDP Receive/1 -> Reshape/1
  Reshape/1 -> inverse_jacobian/1

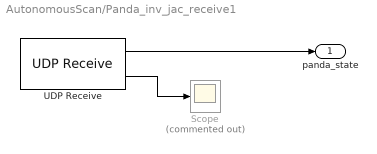
== system AutonomousScan/Panda_inv_jac_receive1 ==
  Scope : Scope  Commented=on
  UDP Receive : dspnetwork/UDP Receive  localURL='0.0.0.0'  localPort=30030  remoteURL='0.0.0.0'  remotePort=-1  recvBufferSize=40  dims=1  signalDatatype=uint8  isComplex=off  isVarSize=off  showBlockingTime=off  blockingTime=0  sampletime=0.001  blockPlatform=[]
      settings: SourceProductName=Simulink
  panda_state : Outport
  wires:
  UDP Receive/2 -> Scope/1
  UDP Receive/1 -> panda_state/1

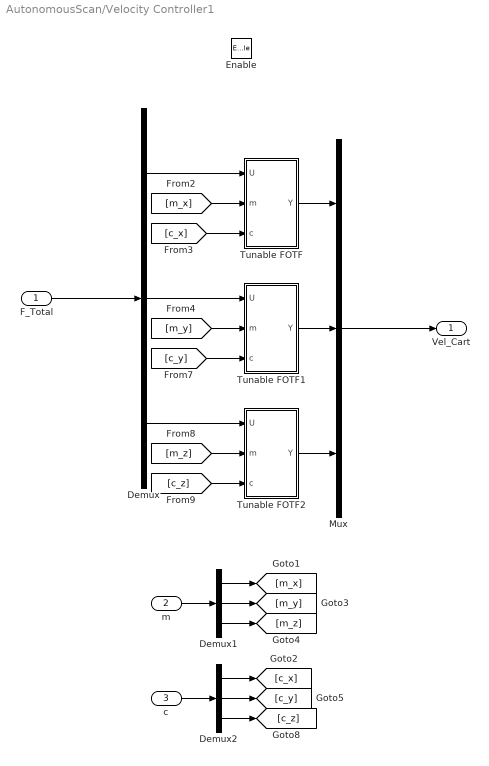
== system AutonomousScan/Velocity Controller1 ==
  F_Total : Inport
  m : Inport  Port=2
  c : Inport  Port=3
  Enable : EnablePort
  Demux : Demux  Outputs=3
  Demux1 : Demux  Outputs=3
  Demux2 : Demux  Outputs=3
  Mux : Mux  Inputs=3
  Tunable FOTF : Subsystem
  Tunable FOTF1 : Subsystem
  Tunable FOTF2 : Subsystem
  Vel_Cart : Outport
  wires:
  [m_y] -> Tunable FOTF1/2(m)
  [c_x] -> Tunable FOTF/3(c)
  Demux/1 -> Tunable FOTF/1(U)
  Tunable FOTF2/1(Y) -> Mux/3
  [m_z] -> Tunable FOTF2/2(m)
  Mux/1 -> Vel_Cart/1
  [c_y] -> Tunable FOTF1/3(c)
  [m_x] -> Tunable FOTF/2(m)
  [c_z] -> Tunable FOTF2/3(c)
  Tunable FOTF/1(Y) -> Mux/1
  Demux/2 -> Tunable FOTF1/1(U)
  F_Total/1 -> Demux/1
  Tunable FOTF1/1(Y) -> Mux/2
  Demux/3 -> Tunable FOTF2/1(U)
  Demux2/2 -> [c_y]
  Demux1/2 -> [m_y]
  c/1 -> Demux2/1
  m/1 -> Demux1/1
  Demux2/1 -> [c_x]
  Demux1/1 -> [m_x]
  Demux1/3 -> [m_z]
  Demux2/3 -> [c_z]

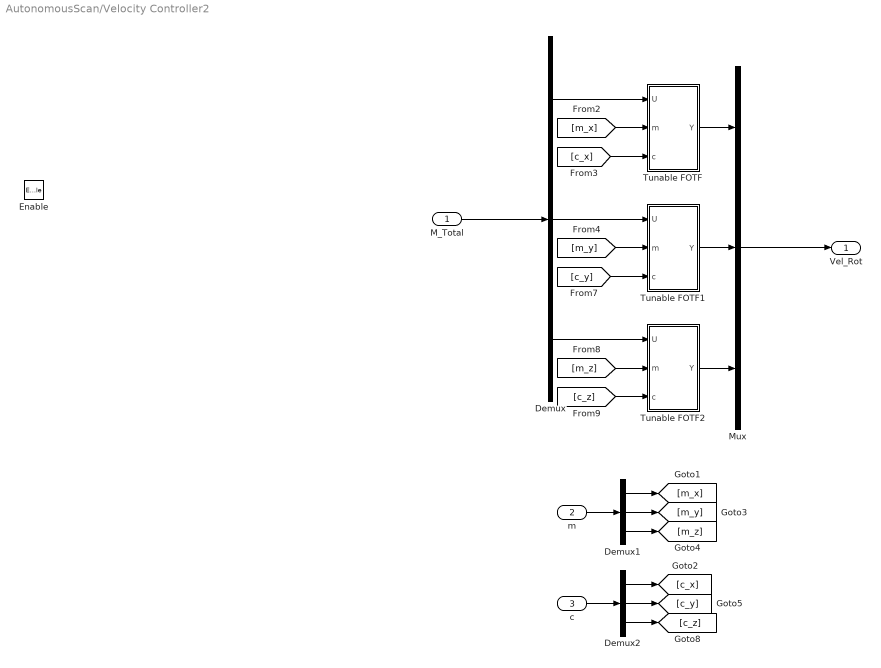
== system AutonomousScan/Velocity Controller2 ==
  M_Total : Inport
  m : Inport  Port=2
  c : Inport  Port=3
  Enable : EnablePort
  Demux : Demux  Outputs=3
  Demux1 : Demux  Outputs=3
  Demux2 : Demux  Outputs=3
  Mux : Mux  Inputs=3
  Tunable FOTF : Subsystem
  Tunable FOTF1 : Subsystem
  Tunable FOTF2 : Subsystem
  Vel_Rot : Outport
  wires:
  [m_y] -> Tunable FOTF1/2(m)
  [c_x] -> Tunable FOTF/3(c)
  Demux/1 -> Tunable FOTF/1(U)
  Tunable FOTF2/1(Y) -> Mux/3
  [m_z] -> Tunable FOTF2/2(m)
  Mux/1 -> Vel_Rot/1
  [c_y] -> Tunable FOTF1/3(c)
  [m_x] -> Tunable FOTF/2(m)
  [c_z] -> Tunable FOTF2/3(c)
  Tunable FOTF/1(Y) -> Mux/1
  Demux/2 -> Tunable FOTF1/1(U)
  M_Total/1 -> Demux/1
  Tunable FOTF1/1(Y) -> Mux/2
  Demux/3 -> Tunable FOTF2/1(U)
  Demux2/2 -> [c_y]
  Demux1/2 -> [m_y]
  c/1 -> Demux2/1
  m/1 -> Demux1/1
  Demux2/1 -> [c_x]
  Demux1/1 -> [m_x]
  Demux1/3 -> [m_z]
  Demux2/3 -> [c_z]

== system AutonomousScan/joy_state_receive1 ==
  Scope : Scope  Commented=on
  UDP Receive : dspnetwork/UDP Receive  localURL='0.0.0.0'  localPort=33333  remoteURL='0.0.0.0'  remotePort=-1  recvBufferSize=840  dims=21  signalDatatype=single  isComplex=off  isVarSize=off  showBlockingTime=off  blockingTime=0  sampletime=0.001  blockPlatform=[]
      settings: SourceProductName=Simulink
  "joy_state " : Outport
  wires:
  UDP Receive/2 -> Scope/1
  UDP Receive/1 -> "joy_state "/1

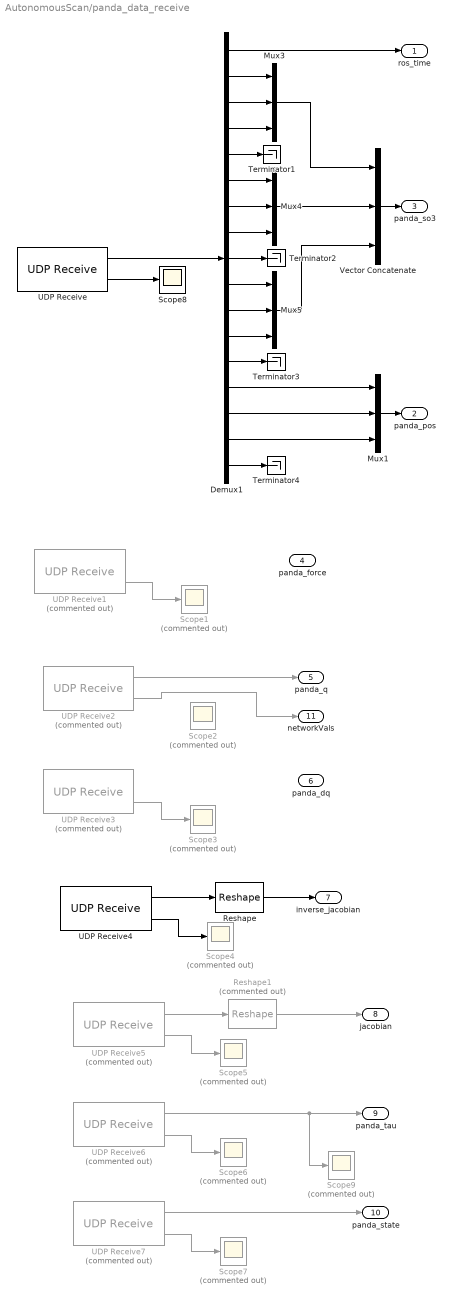
== system AutonomousScan/panda_data_receive ==
  Demux1 : Demux  Outputs=17
  Mux{1,3..5} (4 alike) : Mux  Inputs=3
  Reshape : Reshape  OutputDimensionality=Customize  OutputDimensions=[7,6]
  Reshape1 : Reshape  Commented=on  OutputDimensionality=Customize  OutputDimensions=[7,6]
  Scope{1..7,9} (8 alike) : Scope  Commented=on
  Scope8 : Scope
  Terminator{1..4} (4 alike) : Terminator
  UDP Receive : dspnetwork/UDP Receive  localURL='0.0.0.0'  localPort=30001  remoteURL='127.0.0.1'  remotePort=-1  recvBufferSize=4096  dims=17  signalDatatype=double  isComplex=off  isVarSize=off  showBlockingTime=off  blockingTime=0  sampletime=0.001  blockPlatform=[]
      settings: SourceProductName=Simulink
  UDP Receive1 : dspnetwork/UDP Receive  Commented=on  localURL='0.0.0.0'  localPort=30002  remoteURL='0.0.0.0'  remotePort=-1  recvBufferSize=48  dims=6  signalDatatype=double  isComplex=off  isVarSize=off  showBlockingTime=off  blockingTime=0  sampletime=0.001  blockPlatform=[]
      settings: SourceProductName=Simulink
  UDP Receive2 : dspnetwork/UDP Receive  Commented=on  localURL='0.0.0.0'  localPort=30003  remoteURL='0.0.0.0'  remotePort=-1  recvBufferSize=56  dims=7  signalDatatype=double  isComplex=off  isVarSize=off  showBlockingTime=off  blockingTime=0  sampletime=0.001  blockPlatform=[]
      settings: SourceProductName=Simulink
  UDP Receive3 : dspnetwork/UDP Receive  Commented=on  localURL='0.0.0.0'  localPort=30004  remoteURL='0.0.0.0'  remotePort=-1  recvBufferSize=56  dims=7  signalDatatype=double  isComplex=off  isVarSize=off  showBlockingTime=off  blockingTime=0  sampletime=0.001  blockPlatform=[]
      settings: SourceProductName=Simulink
  UDP Receive4 : dspnetwork/UDP Receive  localURL='0.0.0.0'  localPort=30005  remoteURL='0.0.0.0'  remotePort=-1  recvBufferSize=3360  dims=42  signalDatatype=double  isComplex=off  isVarSize=off  showBlockingTime=off  blockingTime=0  sampletime=0.001  blockPlatform=[]
      settings: SourceProductName=Simulink
  UDP Receive5 : dspnetwork/UDP Receive  Commented=on  localURL='0.0.0.0'  localPort=30006  remoteURL='0.0.0.0'  remotePort=-1  recvBufferSize=3360  dims=42  signalDatatype=double  isComplex=off  isVarSize=off  showBlockingTime=off  blockingTime=0  sampletime=0.001  blockPlatform=[]
      settings: SourceProductName=Simulink
  UDP Receive6 : dspnetwork/UDP Receive  Commented=on  localURL='0.0.0.0'  localPort=30010  remoteURL='0.0.0.0'  remotePort=-1  recvBufferSize=56  dims=7  signalDatatype=double  isComplex=off  isVarSize=off  showBlockingTime=off  blockingTime=0  sampletime=0.001  blockPlatform=[]
      settings: SourceProductName=Simulink
  UDP Receive7 : dspnetwork/UDP Receive  Commented=on  localURL='0.0.0.0'  localPort=30030  remoteURL='0.0.0.0'  remotePort=-1  recvBufferSize=40  dims=1  signalDatatype=uint8  isComplex=off  isVarSize=off  showBlockingTime=off  blockingTime=0  sampletime=0.001  blockPlatform=[]
      settings: SourceProductName=Simulink
  Vector Concatenate : Concatenate  NumInputs=3  Mode=Multidimensional array  ConcatenateDimension=2
  ros_time : Outport
  panda_pos : Outport  Port=2
  panda_so3 : Outport  Port=3
  panda_force : Outport  Port=4
  panda_q : Outport  Port=5
  panda_dq : Outport  Port=6
  inverse_jacobian : Outport  Port=7
  jacobian : Outport  Port=8
  panda_tau : Outport  Port=9
  panda_state : Outport  Port=10
  networkVals : Outport  Port=11
  wires:
  Mux1/1 -> panda_pos/1
  Demux1/6 -> Mux4/1
  Mux3/1 -> Vector Concatenate/1
  Demux1/10 -> Mux5/1
  Demux1/7 -> Mux4/2
  Demux1/12 -> Mux5/3
  Demux1/16 -> Mux1/3
  Demux1/9 -> Terminator2/1
  Demux1/4 -> Mux3/3
  Demux1/15 -> Mux1/2
  Demux1/5 -> Terminator1/1
  Demux1/2 -> Mux3/1
  Demux1/3 -> Mux3/2
  Demux1/1 -> ros_time/1
  Demux1/14 -> Mux1/1
  Mux4/1 -> Vector Concatenate/2
  Demux1/8 -> Mux4/3
  Demux1/11 -> Mux5/2
  Vector Concatenate/1 -> panda_so3/1
  Demux1/13 -> Terminator3/1
  Demux1/17 -> Terminator4/1
  Mux5/1 -> Vector Concatenate/3
  UDP Receive1/2 -> Scope1/1
  UDP Receive2/1 -> panda_q/1
  UDP Receive3/2 -> Scope3/1
  Reshape/1 -> inverse_jacobian/1
  UDP Receive4/2 -> Scope4/1
  UDP Receive4/1 -> Reshape/1
  Reshape1/1 -> jacobian/1
  UDP Receive5/1 -> Reshape1/1
  UDP Receive5/2 -> Scope5/1
  UDP Receive6/1 -> Scope9/1, panda_tau/1
  UDP Receive6/2 -> Scope6/1
  UDP Receive7/1 -> panda_state/1
  UDP Receive7/2 -> Scope7/1
  UDP Receive2/2 -> networkVals/1
  UDP Receive/2 -> Scope8/1
  UDP Receive/1 -> Demux1/1

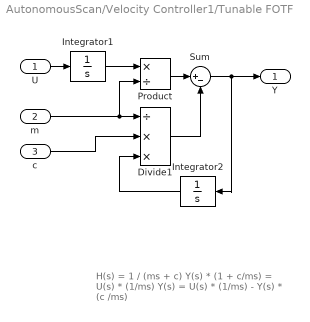
== system AutonomousScan/Velocity Controller1/Tunable FOTF ==
  note: H(s) = 1 / (ms + c)
      | Y(s) * (1 + c/ms) = U(s) * (1/ms)
      | Y(s) = U(s) * (1/ms) - Y(s) * (c /ms)
  U : Inport
  m : Inport  Port=2
  c : Inport  Port=3
  Divide1 : Product  Inputs=/**
  Integrator1 : Integrator
  Integrator2 : Integrator
  Product : Product  Inputs=*/
  Sum : Sum  Inputs=|+-
  Y : Outport
  wires:
  U/1 -> Integrator1/1
  Integrator1/1 -> Product/1
  m/1 -> Divide1/1, Product/2
  Product/1 -> Sum/1
  Sum/1 -> Integrator2/1, Y/1
  c/1 -> Divide1/2
  Divide1/1 -> Sum/2
  Integrator2/1 -> Divide1/3

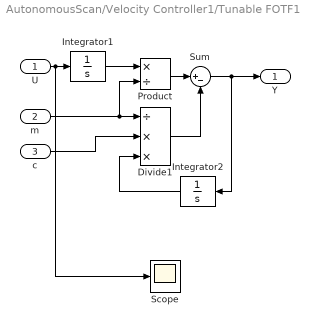
== system AutonomousScan/Velocity Controller1/Tunable FOTF1 ==
  U : Inport
  m : Inport  Port=2
  c : Inport  Port=3
  Divide1 : Product  Inputs=/**
  Integrator1 : Integrator
  Integrator2 : Integrator
  Product : Product  Inputs=*/
  Scope : Scope
  Sum : Sum  Inputs=|+-
  Y : Outport
  wires:
  U/1 -> Scope/1, Integrator1/1
  Integrator1/1 -> Product/1
  m/1 -> Divide1/1, Product/2
  Product/1 -> Sum/1
  Sum/1 -> Integrator2/1, Y/1
  c/1 -> Divide1/2
  Divide1/1 -> Sum/2
  Integrator2/1 -> Divide1/3

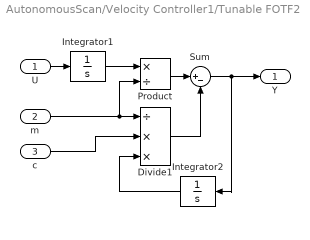
== system AutonomousScan/Velocity Controller1/Tunable FOTF2 ==
  U : Inport
  m : Inport  Port=2
  c : Inport  Port=3
  Divide1 : Product  Inputs=/**
  Integrator1 : Integrator
  Integrator2 : Integrator
  Product : Product  Inputs=*/
  Sum : Sum  Inputs=|+-
  Y : Outport
  wires:
  U/1 -> Integrator1/1
  Integrator1/1 -> Product/1
  m/1 -> Divide1/1, Product/2
  Product/1 -> Sum/1
  Sum/1 -> Integrator2/1, Y/1
  c/1 -> Divide1/2
  Divide1/1 -> Sum/2
  Integrator2/1 -> Divide1/3

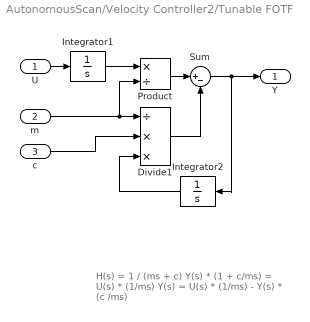
== system AutonomousScan/Velocity Controller2/Tunable FOTF ==
  note: H(s) = 1 / (ms + c)
      | Y(s) * (1 + c/ms) = U(s) * (1/ms)
      | Y(s) = U(s) * (1/ms) - Y(s) * (c /ms)
  U : Inport
  m : Inport  Port=2
  c : Inport  Port=3
  Divide1 : Product  Inputs=/**
  Integrator1 : Integrator
  Integrator2 : Integrator
  Product : Product  Inputs=*/
  Sum : Sum  Inputs=|+-
  Y : Outport
  wires:
  U/1 -> Integrator1/1
  Integrator1/1 -> Product/1
  m/1 -> Divide1/1, Product/2
  Product/1 -> Sum/1
  Sum/1 -> Integrator2/1, Y/1
  c/1 -> Divide1/2
  Divide1/1 -> Sum/2
  Integrator2/1 -> Divide1/3

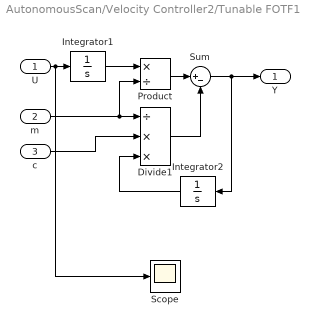
== system AutonomousScan/Velocity Controller2/Tunable FOTF1 ==
  U : Inport
  m : Inport  Port=2
  c : Inport  Port=3
  Divide1 : Product  Inputs=/**
  Integrator1 : Integrator
  Integrator2 : Integrator
  Product : Product  Inputs=*/
  Scope : Scope
  Sum : Sum  Inputs=|+-
  Y : Outport
  wires:
  U/1 -> Scope/1, Integrator1/1
  Integrator1/1 -> Product/1
  m/1 -> Divide1/1, Product/2
  Product/1 -> Sum/1
  Sum/1 -> Integrator2/1, Y/1
  c/1 -> Divide1/2
  Divide1/1 -> Sum/2
  Integrator2/1 -> Divide1/3

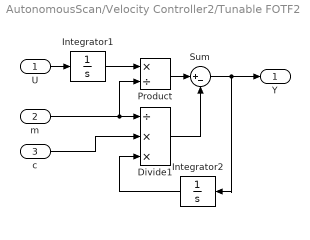
== system AutonomousScan/Velocity Controller2/Tunable FOTF2 ==
  U : Inport
  m : Inport  Port=2
  c : Inport  Port=3
  Divide1 : Product  Inputs=/**
  Integrator1 : Integrator
  Integrator2 : Integrator
  Product : Product  Inputs=*/
  Sum : Sum  Inputs=|+-
  Y : Outport
  wires:
  U/1 -> Integrator1/1
  Integrator1/1 -> Product/1
  m/1 -> Divide1/1, Product/2
  Product/1 -> Sum/1
  Sum/1 -> Integrator2/1, Y/1
  c/1 -> Divide1/2
  Divide1/1 -> Sum/2
  Integrator2/1 -> Divide1/3

== matlab function AutonomousScan/MATLAB Function1 ==
  data: u input; y output
function y = fcn(u)
    for i = 1:3
        if u(i)>pi
            u(i) = u(i)-(2*pi)
        elseif u(i)<-pi
            u(i) = u(i)+(2*pi)
        end
    end
y = u;

== matlab function AutonomousScan/MATLAB Function2 ==
  data: x input; x_rot output; R input
function x_rot = rot(x,R)
%#codegen
x_rot = R*x;
end

== matlab function AutonomousScan/MATLAB Function3 ==
  data: f_des input; f_err output; f_act input; bias_good input
function f_err  = f_err_z(f_des, f_act, bias_good)
%#codegen
f_err = zeros(3,1);
if bias_good == false
    return
elseif bias_good == true    
    f_err(3) = f_des - f_act(3);
end

== matlab function AutonomousScan/MATLAB Function4 ==
  data: X input; arad input; brad input; grad input; X_t output
function X_t  = rot(X,arad,brad,grad)
%#codegen
Rz = [cos(arad) -sin(arad) 0; sin(arad) cos(arad) 0; 0 0 1];
Ry = [cos(brad) 0 sin(brad); 0 1 0; -sin(brad) 0 cos(brad)];
Rx = [1 0 0; 0 cos(grad) -sin(grad); 0 sin(grad) cos(grad)];
T = Rz * Ry * Rx;
T = -T;
X_t = T*X;

== matlab function AutonomousScan/MATLAB Function ==
  data: x input; x_rot output; R input
function x_rot = rot(x,R)
%#codegen
x_rot = R*x;
end

== matlab function AutonomousScan/MATLAB Function5 ==
  data: forceMeasure input; bias output; forceBiasGood output; currentPos input; desiredPos input
function [bias, forceBiasGood] = forceBias(forceMeasure,currentPos,desiredPos)
persistent n force_sensor_data
data_limit = 5000;
pos_max_error = 0.0007;

if isempty(force_sensor_data)
    force_sensor_data = zeros(6,data_limit);
end

if isempty(n)
    n = 1;
end

errPos = sum(abs(currentPos - desiredPos));
if(errPos <= pos_max_error && n <= data_limit)
    %if(n <= data_limit && biasPosGood)
    if(sum(abs(forceMeasure)) ~= 0)
        force_sensor_data(:,n) = forceMeasure;
        n = n + 1;
    end
end

bias = zeros(6,1);
forceBiasGood = false;

if(n > data_limit)
    force_sensor_data_means = mean(force_sensor_data,2);
    bias(:) = force_sensor_data_means;
    forceBiasGood = true;
end

== matlab function AutonomousScan/MATLAB Function6 ==
  data: X input; X_t output; arad input; brad input; grad input
function X_t  = rot(X,arad,brad,grad)
%#codegen
Rz = [cos(arad) -sin(arad) 0; sin(arad) cos(arad) 0; 0 0 1];
Ry = [cos(brad) 0 sin(brad); 0 1 0; -sin(brad) 0 cos(brad)];
Rx = [1 0 0; 0 cos(grad) -sin(grad); 0 sin(grad) cos(grad)];
T = Rz * Ry * Rx;
T = -T; %force sensor was installed upside down
X_t = T*X;

== matlab function AutonomousScan/MATLAB Function7 ==
  data: X input; X_t output; arad input; brad input; grad input
function X_t  = rot(X,arad,brad,grad)
%#codegen
Rz = [cos(arad) -sin(arad) 0; sin(arad) cos(arad) 0; 0 0 1];
Ry = [cos(brad) 0 sin(brad); 0 1 0; -sin(brad) 0 cos(brad)];
Rx = [1 0 0; 0 cos(grad) -sin(grad); 0 sin(grad) cos(grad)];
T = Rz * Ry * Rx;
T(3,3) = -T(3,3);
X_t = T*X;

== matlab function AutonomousScan/New Phantom ==
  settings: updateMethod=DISCRETE
  data: shutter_fb input; pos_des output; current_pos input; record_data output; measured_force input; bias_good input; shutter output; pnts output; scan_complete output
function [pos_des, record_data, shutter, pnts, scan_complete] = fcn(shutter_fb, current_pos, measured_force, bias_good)
persistent k contact_made pnt shutter_pass scan_fin

if isempty(k)
    k = 1;
end

if isempty(contact_made)
    contact_made = false;
end

if isempty(pnt)
    pnt = 1;
end

if isempty(shutter_pass)
    shutter_pass = 0;
end

if isempty(scan_fin)
    scan_fin = 0;
end


%constants - previously y was [0.085 0.005] previously x was [0.483 0.458]
%number of trajectory points must be even
trajectory = [0.483 0.000 0.175;
    
% 0.483 0.06 0.175

% 0.483 0.000 0.175

0.46 0.000 0.175

0.46 0.06 0.175

0.46 0.06 0.175];

pos_max_error_fine = 0.0001;
x_dist = 0.00125; %(0.475-0.425)/25
contact_force = -1.1;
num_points = ceil(abs(max(trajectory(:,2))-min(trajectory(:,2)))/x_dist)+1;

smooth_traj = repmat(trajectory(1,:), num_points, 1); 
shutter = 0;

%set contact flag by measuring z force
if bias_good == true && measured_force(3) <= contact_force
    contact_made = true;
end

%selective recording
% if contact_made == true && mod(k,2) == 0
if mod(k,2) == 0
    record_data = 1;
else
    record_data = 0;
end

%generates trajectory between adjecent points
if record_data == 1
    if trajectory(k,2) > trajectory(k+1,2)
        x_dist = -x_dist;
    end
        
    for t = 1:num_points
        smooth_traj(t,:) = [trajectory(k,1) trajectory(k,2)+(t-1)*x_dist trajectory(k,3)]; 
    end

elseif contact_made == true && record_data == 0 
    for t = 1:num_points
        smooth_traj(t,:) = trajectory(k+1,:);
    end
end

%send desired coordinates to robot
pos_des = smooth_traj(pnt, :).';

err_pos_fine = sum(abs(current_pos(1:2,1) - pos_des(1:2,1)));
if record_data == 1 && err_pos_fine <= pos_max_error_fine

    shutter_pass = 1; 
    
    if shutter_fb == 1
        pnt = pnt + 1;
        if pnt > num_points
            pnt = 1;
        end
        shutter_pass = 0;
    end
end

%checks if vector end point has been reached
err_pos = sum(abs(current_pos(1:2,1) - trajectory(k+1,1:2).'));
if contact_made == true && err_pos <= pos_max_error_fine

    shutter_pass = 1;
    if shutter_fb == 1
        %switches to next set of adjacent points
        k = k + 1;
        
        %checks if end of trajectory
        if k == size(trajectory, 1)
            k = size(trajectory, 1) - 1;
            scan_fin = 1;
        end
        
        %reset counter
        pnt = 1;
        shutter_pass = 0;
    end
    
    if k == size(trajectory, 1) - 1
        shutter_pass = 0;
    end
end

if shutter_pass == 1 && shutter_fb ~= 1
    shutter = 1;
    
end



pnts = pnt;
scan_complete = scan_fin;
end

== matlab function AutonomousScan/MATLAB Function8 ==
  data: x input; x_rot output; R input
function x_rot = rot(x,R)
%#codegen
x_rot = R*x;
end

== matlab function AutonomousScan/in general2 ==
  data: R input; arad output; brad output; grad output
function [arad,brad,grad] = so3_to_rpy(R)
sy = sqrt(R(3,2)^2 + R(3,3)^2);
if sy > eps
    % non singular
    arad = atan2(R(3,2),R(3,3));
    brad = atan2(-R(3,1),sy);
    grad = atan2(R(2,1),R(1,1));
else
    % singular
    arad = atan2(-R(2,3),R(2,2));
    brad = atan2(-R(3,1),sy);
    grad = 0;
end
end
